simulink model "Day21"  (R2024b)
settings: Solver=VariableStepAuto  StartTime=0.0  StopTime=10.0  RelTol=1e-3
settings Model: Creator=jun_mac  LastModifiedBy=jun_mac

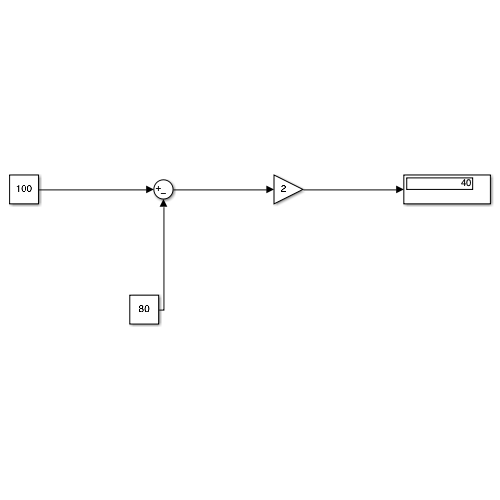
[thumbnail: Simulink's stored preview of the top-level diagram]
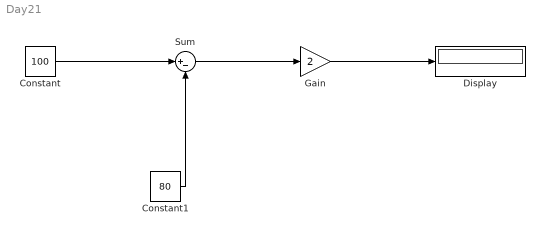
== system Day21 ==
  Constant : Constant  Value=100
  Constant1 : Constant  Value=80
  Display : Display
  Gain : Gain  Gain=2
  Sum : Sum  Inputs=|+-
  wires:
  Constant1/1 -> Sum/2
  Constant/1 -> Sum/1
  Sum/1 -> Gain/1
  Gain/1 -> Display/1
